simulink model "c00003M_harness"  (R2018a)
settings: Solver=FixedStepAuto  StartTime=0.0  StopTime=300  FixedStep=0.1  RelTol=1e-3
undefined symbols (not defined in the file): A1, hmax, PriorityTank, R1, R2, sigbuilder_block
(part 6 of 44)

== system c00003M_harness/M062 ==
  note: VALUES
      | ---------------------------------
      | ControlType = 1 | 2 | 3
      | FillTank = 0 | 1
      | EmptyTank = 0 | 1
      | ManualReference between 0 and 1
      | Tempreature between 0 and 100
      | EmergencyButton = 0 | 1
      | LiquidLevel between 0 and 1 (hmax)
  note: Inputs For Tank2
  note: NAMES
      | --------------------------------------------
      | CT1 = ControlType Tank 1
      | F1 = Fill Tank 1
      | E1 = Empty Tank 1
      | MR1 = Manual Reference Tank1
      | T1 = Temperature Tank 1
      | EB1 = Emergency Button Tank 1
      | LL1 = Liquid Level 1
  note: Inputs For Tank3
  note: Inputs For Tank1
  CT1 : Inport
  F1 : Inport  Port=2
  E1 : Inport  Port=3
  MR1 : Inport  Port=4
  T1 : Inport  Port=5
  EB1 : Inport  Port=6
  CT2 : Inport  Port=7
  F2 : Inport  Port=8
  E2 : Inport  Port=9
  MR2 : Inport  Port=10
  T2 : Inport  Port=11
  EB2 : Inport  Port=12
  Tank1 : Subsystem
  Tank2 : Subsystem
  LL1 : Outport
  LL2 : Outport  Port=2
  wires:
  EB1/1 -> Tank1/6(EB1)
  Tank2/1(LL2) -> LL2/1, Tank1/7(LL2)
  EB2/1 -> Tank2/6(EB2)
  CT2/1 -> Tank2/1(CT2)
  MR1/1 -> Tank1/4(MR1)
  T1/1 -> Tank1/5(T1)
  Tank1/1(LL1) -> LL1/1, Tank2/7(LL1)
  F2/1 -> Tank2/2(F2)
  E2/1 -> Tank2/3(E2)
  F1/1 -> Tank1/2(F1)
  E1/1 -> Tank1/3(E1)
  T2/1 -> Tank2/5(T2)
  CT1/1 -> Tank1/1(CT1)
  MR2/1 -> Tank2/4(MR2)

== system c00003M_harness/M063 ==
  note: VALUES
      | ---------------------------------
      | ControlType = 1 | 2 | 3
      | FillTank = 0 | 1
      | EmptyTank = 0 | 1
      | ManualReference between 0 and 1
      | Tempreature between 0 and 100
      | EmergencyButton = 0 | 1
      | LiquidLevel between 0 and 1 (hmax)
  note: Inputs For Tank2
  note: NAMES
      | --------------------------------------------
      | CT1 = ControlType Tank 1
      | F1 = Fill Tank 1
      | E1 = Empty Tank 1
      | MR1 = Manual Reference Tank1
      | T1 = Temperature Tank 1
      | EB1 = Emergency Button Tank 1
      | LL1 = Liquid Level 1
  note: Inputs For Tank3
  note: Inputs For Tank1
  CT1 : Inport
  F1 : Inport  Port=2
  E1 : Inport  Port=3
  MR1 : Inport  Port=4
  T1 : Inport  Port=5
  EB1 : Inport  Port=6
  CT2 : Inport  Port=7
  F2 : Inport  Port=8
  E2 : Inport  Port=9
  MR2 : Inport  Port=10
  T2 : Inport  Port=11
  EB2 : Inport  Port=12
  Tank1 : Subsystem
  Tank2 : Subsystem
  LL1 : Outport
  LL2 : Outport  Port=2
  wires:
  EB1/1 -> Tank1/6(EB1)
  Tank2/1(LL2) -> LL2/1, Tank1/7(LL2)
  EB2/1 -> Tank2/6(EB2)
  CT2/1 -> Tank2/1(CT2)
  MR1/1 -> Tank1/4(MR1)
  T1/1 -> Tank1/5(T1)
  Tank1/1(LL1) -> LL1/1, Tank2/7(LL1)
  F2/1 -> Tank2/2(F2)
  E2/1 -> Tank2/3(E2)
  F1/1 -> Tank1/2(F1)
  E1/1 -> Tank1/3(E1)
  T2/1 -> Tank2/5(T2)
  CT1/1 -> Tank1/1(CT1)
  MR2/1 -> Tank2/4(MR2)

== system c00003M_harness/M064 ==
  note: VALUES
      | ---------------------------------
      | ControlType = 1 | 2 | 3
      | FillTank = 0 | 1
      | EmptyTank = 0 | 1
      | ManualReference between 0 and 1
      | Tempreature between 0 and 100
      | EmergencyButton = 0 | 1
      | LiquidLevel between 0 and 1 (hmax)
  note: Inputs For Tank2
  note: NAMES
      | --------------------------------------------
      | CT1 = ControlType Tank 1
      | F1 = Fill Tank 1
      | E1 = Empty Tank 1
      | MR1 = Manual Reference Tank1
      | T1 = Temperature Tank 1
      | EB1 = Emergency Button Tank 1
      | LL1 = Liquid Level 1
  note: Inputs For Tank3
  note: Inputs For Tank1
  CT1 : Inport
  F1 : Inport  Port=2
  E1 : Inport  Port=3
  MR1 : Inport  Port=4
  T1 : Inport  Port=5
  EB1 : Inport  Port=6
  CT2 : Inport  Port=7
  F2 : Inport  Port=8
  E2 : Inport  Port=9
  MR2 : Inport  Port=10
  T2 : Inport  Port=11
  EB2 : Inport  Port=12
  Tank1 : Subsystem
  Tank2 : Subsystem
  LL1 : Outport
  LL2 : Outport  Port=2
  wires:
  EB1/1 -> Tank1/6(EB1)
  Tank2/1(LL2) -> LL2/1, Tank1/7(LL2)
  EB2/1 -> Tank2/6(EB2)
  CT2/1 -> Tank2/1(CT2)
  MR1/1 -> Tank1/4(MR1)
  T1/1 -> Tank1/5(T1)
  Tank1/1(LL1) -> LL1/1, Tank2/7(LL1)
  F2/1 -> Tank2/2(F2)
  E2/1 -> Tank2/3(E2)
  F1/1 -> Tank1/2(F1)
  E1/1 -> Tank1/3(E1)
  T2/1 -> Tank2/5(T2)
  CT1/1 -> Tank1/1(CT1)
  MR2/1 -> Tank2/4(MR2)

== system c00003M_harness/M065 ==
  note: VALUES
      | ---------------------------------
      | ControlType = 1 | 2 | 3
      | FillTank = 0 | 1
      | EmptyTank = 0 | 1
      | ManualReference between 0 and 1
      | Tempreature between 0 and 100
      | EmergencyButton = 0 | 1
      | LiquidLevel between 0 and 1 (hmax)
  note: Inputs For Tank2
  note: NAMES
      | --------------------------------------------
      | CT1 = ControlType Tank 1
      | F1 = Fill Tank 1
      | E1 = Empty Tank 1
      | MR1 = Manual Reference Tank1
      | T1 = Temperature Tank 1
      | EB1 = Emergency Button Tank 1
      | LL1 = Liquid Level 1
  note: Inputs For Tank3
  note: Inputs For Tank1
  CT1 : Inport
  F1 : Inport  Port=2
  E1 : Inport  Port=3
  MR1 : Inport  Port=4
  T1 : Inport  Port=5
  EB1 : Inport  Port=6
  CT2 : Inport  Port=7
  F2 : Inport  Port=8
  E2 : Inport  Port=9
  MR2 : Inport  Port=10
  T2 : Inport  Port=11
  EB2 : Inport  Port=12
  Tank1 : Subsystem
  Tank2 : Subsystem
  LL1 : Outport
  LL2 : Outport  Port=2
  wires:
  EB1/1 -> Tank1/6(EB1)
  Tank2/1(LL2) -> LL2/1, Tank1/7(LL2)
  EB2/1 -> Tank2/6(EB2)
  CT2/1 -> Tank2/1(CT2)
  MR1/1 -> Tank1/4(MR1)
  T1/1 -> Tank1/5(T1)
  Tank1/1(LL1) -> LL1/1, Tank2/7(LL1)
  F2/1 -> Tank2/2(F2)
  E2/1 -> Tank2/3(E2)
  F1/1 -> Tank1/2(F1)
  E1/1 -> Tank1/3(E1)
  T2/1 -> Tank2/5(T2)
  CT1/1 -> Tank1/1(CT1)
  MR2/1 -> Tank2/4(MR2)

== system c00003M_harness/M066 ==
  note: VALUES
      | ---------------------------------
      | ControlType = 1 | 2 | 3
      | FillTank = 0 | 1
      | EmptyTank = 0 | 1
      | ManualReference between 0 and 1
      | Tempreature between 0 and 100
      | EmergencyButton = 0 | 1
      | LiquidLevel between 0 and 1 (hmax)
  note: Inputs For Tank2
  note: NAMES
      | --------------------------------------------
      | CT1 = ControlType Tank 1
      | F1 = Fill Tank 1
      | E1 = Empty Tank 1
      | MR1 = Manual Reference Tank1
      | T1 = Temperature Tank 1
      | EB1 = Emergency Button Tank 1
      | LL1 = Liquid Level 1
  note: Inputs For Tank3
  note: Inputs For Tank1
  CT1 : Inport
  F1 : Inport  Port=2
  E1 : Inport  Port=3
  MR1 : Inport  Port=4
  T1 : Inport  Port=5
  EB1 : Inport  Port=6
  CT2 : Inport  Port=7
  F2 : Inport  Port=8
  E2 : Inport  Port=9
  MR2 : Inport  Port=10
  T2 : Inport  Port=11
  EB2 : Inport  Port=12
  Tank1 : Subsystem
  Tank2 : Subsystem
  LL1 : Outport
  LL2 : Outport  Port=2
  wires:
  EB1/1 -> Tank1/6(EB1)
  Tank2/1(LL2) -> LL2/1, Tank1/7(LL2)
  EB2/1 -> Tank2/6(EB2)
  CT2/1 -> Tank2/1(CT2)
  MR1/1 -> Tank1/4(MR1)
  T1/1 -> Tank1/5(T1)
  Tank1/1(LL1) -> LL1/1, Tank2/7(LL1)
  F2/1 -> Tank2/2(F2)
  E2/1 -> Tank2/3(E2)
  F1/1 -> Tank1/2(F1)
  E1/1 -> Tank1/3(E1)
  T2/1 -> Tank2/5(T2)
  CT1/1 -> Tank1/1(CT1)
  MR2/1 -> Tank2/4(MR2)

== system c00003M_harness/M067 ==
  note: VALUES
      | ---------------------------------
      | ControlType = 1 | 2 | 3
      | FillTank = 0 | 1
      | EmptyTank = 0 | 1
      | ManualReference between 0 and 1
      | Tempreature between 0 and 100
      | EmergencyButton = 0 | 1
      | LiquidLevel between 0 and 1 (hmax)
  note: Inputs For Tank2
  note: NAMES
      | --------------------------------------------
      | CT1 = ControlType Tank 1
      | F1 = Fill Tank 1
      | E1 = Empty Tank 1
      | MR1 = Manual Reference Tank1
      | T1 = Temperature Tank 1
      | EB1 = Emergency Button Tank 1
      | LL1 = Liquid Level 1
  note: Inputs For Tank3
  note: Inputs For Tank1
  CT1 : Inport
  F1 : Inport  Port=2
  E1 : Inport  Port=3
  MR1 : Inport  Port=4
  T1 : Inport  Port=5
  EB1 : Inport  Port=6
  CT2 : Inport  Port=7
  F2 : Inport  Port=8
  E2 : Inport  Port=9
  MR2 : Inport  Port=10
  T2 : Inport  Port=11
  EB2 : Inport  Port=12
  Tank1 : Subsystem
  Tank2 : Subsystem
  LL1 : Outport
  LL2 : Outport  Port=2
  wires:
  EB1/1 -> Tank1/6(EB1)
  Tank2/1(LL2) -> LL2/1, Tank1/7(LL2)
  EB2/1 -> Tank2/6(EB2)
  CT2/1 -> Tank2/1(CT2)
  MR1/1 -> Tank1/4(MR1)
  T1/1 -> Tank1/5(T1)
  Tank1/1(LL1) -> LL1/1, Tank2/7(LL1)
  F2/1 -> Tank2/2(F2)
  E2/1 -> Tank2/3(E2)
  F1/1 -> Tank1/2(F1)
  E1/1 -> Tank1/3(E1)
  T2/1 -> Tank2/5(T2)
  CT1/1 -> Tank1/1(CT1)
  MR2/1 -> Tank2/4(MR2)

== system c00003M_harness/M068 ==
  note: VALUES
      | ---------------------------------
      | ControlType = 1 | 2 | 3
      | FillTank = 0 | 1
      | EmptyTank = 0 | 1
      | ManualReference between 0 and 1
      | Tempreature between 0 and 100
      | EmergencyButton = 0 | 1
      | LiquidLevel between 0 and 1 (hmax)
  note: Inputs For Tank2
  note: NAMES
      | --------------------------------------------
      | CT1 = ControlType Tank 1
      | F1 = Fill Tank 1
      | E1 = Empty Tank 1
      | MR1 = Manual Reference Tank1
      | T1 = Temperature Tank 1
      | EB1 = Emergency Button Tank 1
      | LL1 = Liquid Level 1
  note: Inputs For Tank3
  note: Inputs For Tank1
  CT1 : Inport
  F1 : Inport  Port=2
  E1 : Inport  Port=3
  MR1 : Inport  Port=4
  T1 : Inport  Port=5
  EB1 : Inport  Port=6
  CT2 : Inport  Port=7
  F2 : Inport  Port=8
  E2 : Inport  Port=9
  MR2 : Inport  Port=10
  T2 : Inport  Port=11
  EB2 : Inport  Port=12
  Tank1 : Subsystem
  Tank2 : Subsystem
  LL1 : Outport
  LL2 : Outport  Port=2
  wires:
  EB1/1 -> Tank1/6(EB1)
  Tank2/1(LL2) -> LL2/1, Tank1/7(LL2)
  EB2/1 -> Tank2/6(EB2)
  CT2/1 -> Tank2/1(CT2)
  MR1/1 -> Tank1/4(MR1)
  T1/1 -> Tank1/5(T1)
  Tank1/1(LL1) -> LL1/1, Tank2/7(LL1)
  F2/1 -> Tank2/2(F2)
  E2/1 -> Tank2/3(E2)
  F1/1 -> Tank1/2(F1)
  E1/1 -> Tank1/3(E1)
  T2/1 -> Tank2/5(T2)
  CT1/1 -> Tank1/1(CT1)
  MR2/1 -> Tank2/4(MR2)

== system c00003M_harness/M069 ==
  note: VALUES
      | ---------------------------------
      | ControlType = 1 | 2 | 3
      | FillTank = 0 | 1
      | EmptyTank = 0 | 1
      | ManualReference between 0 and 1
      | Tempreature between 0 and 100
      | EmergencyButton = 0 | 1
      | LiquidLevel between 0 and 1 (hmax)
  note: Inputs For Tank2
  note: NAMES
      | --------------------------------------------
      | CT1 = ControlType Tank 1
      | F1 = Fill Tank 1
      | E1 = Empty Tank 1
      | MR1 = Manual Reference Tank1
      | T1 = Temperature Tank 1
      | EB1 = Emergency Button Tank 1
      | LL1 = Liquid Level 1
  note: Inputs For Tank3
  note: Inputs For Tank1
  CT1 : Inport
  F1 : Inport  Port=2
  E1 : Inport  Port=3
  MR1 : Inport  Port=4
  T1 : Inport  Port=5
  EB1 : Inport  Port=6
  CT2 : Inport  Port=7
  F2 : Inport  Port=8
  E2 : Inport  Port=9
  MR2 : Inport  Port=10
  T2 : Inport  Port=11
  EB2 : Inport  Port=12
  Tank1 : Subsystem
  Tank2 : Subsystem
  LL1 : Outport
  LL2 : Outport  Port=2
  wires:
  EB1/1 -> Tank1/6(EB1)
  Tank2/1(LL2) -> LL2/1, Tank1/7(LL2)
  EB2/1 -> Tank2/6(EB2)
  CT2/1 -> Tank2/1(CT2)
  MR1/1 -> Tank1/4(MR1)
  T1/1 -> Tank1/5(T1)
  Tank1/1(LL1) -> LL1/1, Tank2/7(LL1)
  F2/1 -> Tank2/2(F2)
  E2/1 -> Tank2/3(E2)
  F1/1 -> Tank1/2(F1)
  E1/1 -> Tank1/3(E1)
  T2/1 -> Tank2/5(T2)
  CT1/1 -> Tank1/1(CT1)
  MR2/1 -> Tank2/4(MR2)

== system c00003M_harness/M070 ==
  note: VALUES
      | ---------------------------------
      | ControlType = 1 | 2 | 3
      | FillTank = 0 | 1
      | EmptyTank = 0 | 1
      | ManualReference between 0 and 1
      | Tempreature between 0 and 100
      | EmergencyButton = 0 | 1
      | LiquidLevel between 0 and 1 (hmax)
  note: Inputs For Tank2
  note: NAMES
      | --------------------------------------------
      | CT1 = ControlType Tank 1
      | F1 = Fill Tank 1
      | E1 = Empty Tank 1
      | MR1 = Manual Reference Tank1
      | T1 = Temperature Tank 1
      | EB1 = Emergency Button Tank 1
      | LL1 = Liquid Level 1
  note: Inputs For Tank3
  note: Inputs For Tank1
  CT1 : Inport
  F1 : Inport  Port=2
  E1 : Inport  Port=3
  MR1 : Inport  Port=4
  T1 : Inport  Port=5
  EB1 : Inport  Port=6
  CT2 : Inport  Port=7
  F2 : Inport  Port=8
  E2 : Inport  Port=9
  MR2 : Inport  Port=10
  T2 : Inport  Port=11
  EB2 : Inport  Port=12
  Tank1 : Subsystem
  Tank2 : Subsystem
  LL1 : Outport
  LL2 : Outport  Port=2
  wires:
  EB1/1 -> Tank1/6(EB1)
  Tank2/1(LL2) -> LL2/1, Tank1/7(LL2)
  EB2/1 -> Tank2/6(EB2)
  CT2/1 -> Tank2/1(CT2)
  MR1/1 -> Tank1/4(MR1)
  T1/1 -> Tank1/5(T1)
  Tank1/1(LL1) -> LL1/1, Tank2/7(LL1)
  F2/1 -> Tank2/2(F2)
  E2/1 -> Tank2/3(E2)
  F1/1 -> Tank1/2(F1)
  E1/1 -> Tank1/3(E1)
  T2/1 -> Tank2/5(T2)
  CT1/1 -> Tank1/1(CT1)
  MR2/1 -> Tank2/4(MR2)

== system c00003M_harness/M071 ==
  note: VALUES
      | ---------------------------------
      | ControlType = 1 | 2 | 3
      | FillTank = 0 | 1
      | EmptyTank = 0 | 1
      | ManualReference between 0 and 1
      | Tempreature between 0 and 100
      | EmergencyButton = 0 | 1
      | LiquidLevel between 0 and 1 (hmax)
  note: Inputs For Tank2
  note: NAMES
      | --------------------------------------------
      | CT1 = ControlType Tank 1
      | F1 = Fill Tank 1
      | E1 = Empty Tank 1
      | MR1 = Manual Reference Tank1
      | T1 = Temperature Tank 1
      | EB1 = Emergency Button Tank 1
      | LL1 = Liquid Level 1
  note: Inputs For Tank3
  note: Inputs For Tank1
  CT1 : Inport
  F1 : Inport  Port=2
  E1 : Inport  Port=3
  MR1 : Inport  Port=4
  T1 : Inport  Port=5
  EB1 : Inport  Port=6
  CT2 : Inport  Port=7
  F2 : Inport  Port=8
  E2 : Inport  Port=9
  MR2 : Inport  Port=10
  T2 : Inport  Port=11
  EB2 : Inport  Port=12
  Tank1 : Subsystem
  Tank2 : Subsystem
  LL1 : Outport
  LL2 : Outport  Port=2
  wires:
  EB1/1 -> Tank1/6(EB1)
  Tank2/1(LL2) -> LL2/1, Tank1/7(LL2)
  EB2/1 -> Tank2/6(EB2)
  CT2/1 -> Tank2/1(CT2)
  MR1/1 -> Tank1/4(MR1)
  T1/1 -> Tank1/5(T1)
  Tank1/1(LL1) -> LL1/1, Tank2/7(LL1)
  F2/1 -> Tank2/2(F2)
  E2/1 -> Tank2/3(E2)
  F1/1 -> Tank1/2(F1)
  E1/1 -> Tank1/3(E1)
  T2/1 -> Tank2/5(T2)
  CT1/1 -> Tank1/1(CT1)
  MR2/1 -> Tank2/4(MR2)

== system c00003M_harness/M072 ==
  note: VALUES
      | ---------------------------------
      | ControlType = 1 | 2 | 3
      | FillTank = 0 | 1
      | EmptyTank = 0 | 1
      | ManualReference between 0 and 1
      | Tempreature between 0 and 100
      | EmergencyButton = 0 | 1
      | LiquidLevel between 0 and 1 (hmax)
  note: Inputs For Tank2
  note: NAMES
      | --------------------------------------------
      | CT1 = ControlType Tank 1
      | F1 = Fill Tank 1
      | E1 = Empty Tank 1
      | MR1 = Manual Reference Tank1
      | T1 = Temperature Tank 1
      | EB1 = Emergency Button Tank 1
      | LL1 = Liquid Level 1
  note: Inputs For Tank3
  note: Inputs For Tank1
  CT1 : Inport
  F1 : Inport  Port=2
  E1 : Inport  Port=3
  MR1 : Inport  Port=4
  T1 : Inport  Port=5
  EB1 : Inport  Port=6
  CT2 : Inport  Port=7
  F2 : Inport  Port=8
  E2 : Inport  Port=9
  MR2 : Inport  Port=10
  T2 : Inport  Port=11
  EB2 : Inport  Port=12
  Tank1 : Subsystem
  Tank2 : Subsystem
  LL1 : Outport
  LL2 : Outport  Port=2
  wires:
  EB1/1 -> Tank1/6(EB1)
  Tank2/1(LL2) -> LL2/1, Tank1/7(LL2)
  EB2/1 -> Tank2/6(EB2)
  CT2/1 -> Tank2/1(CT2)
  MR1/1 -> Tank1/4(MR1)
  T1/1 -> Tank1/5(T1)
  Tank1/1(LL1) -> LL1/1, Tank2/7(LL1)
  F2/1 -> Tank2/2(F2)
  E2/1 -> Tank2/3(E2)
  F1/1 -> Tank1/2(F1)
  E1/1 -> Tank1/3(E1)
  T2/1 -> Tank2/5(T2)
  CT1/1 -> Tank1/1(CT1)
  MR2/1 -> Tank2/4(MR2)

== system c00003M_harness/M073 ==
  note: VALUES
      | ---------------------------------
      | ControlType = 1 | 2 | 3
      | FillTank = 0 | 1
      | EmptyTank = 0 | 1
      | ManualReference between 0 and 1
      | Tempreature between 0 and 100
      | EmergencyButton = 0 | 1
      | LiquidLevel between 0 and 1 (hmax)
  note: Inputs For Tank2
  note: NAMES
      | --------------------------------------------
      | CT1 = ControlType Tank 1
      | F1 = Fill Tank 1
      | E1 = Empty Tank 1
      | MR1 = Manual Reference Tank1
      | T1 = Temperature Tank 1
      | EB1 = Emergency Button Tank 1
      | LL1 = Liquid Level 1
  note: Inputs For Tank3
  note: Inputs For Tank1
  CT1 : Inport
  F1 : Inport  Port=2
  E1 : Inport  Port=3
  MR1 : Inport  Port=4
  T1 : Inport  Port=5
  EB1 : Inport  Port=6
  CT2 : Inport  Port=7
  F2 : Inport  Port=8
  E2 : Inport  Port=9
  MR2 : Inport  Port=10
  T2 : Inport  Port=11
  EB2 : Inport  Port=12
  Tank1 : Subsystem
  Tank2 : Subsystem
  LL1 : Outport
  LL2 : Outport  Port=2
  wires:
  EB1/1 -> Tank1/6(EB1)
  Tank2/1(LL2) -> LL2/1, Tank1/7(LL2)
  EB2/1 -> Tank2/6(EB2)
  CT2/1 -> Tank2/1(CT2)
  MR1/1 -> Tank1/4(MR1)
  T1/1 -> Tank1/5(T1)
  Tank1/1(LL1) -> LL1/1, Tank2/7(LL1)
  F2/1 -> Tank2/2(F2)
  E2/1 -> Tank2/3(E2)
  F1/1 -> Tank1/2(F1)
  E1/1 -> Tank1/3(E1)
  T2/1 -> Tank2/5(T2)
  CT1/1 -> Tank1/1(CT1)
  MR2/1 -> Tank2/4(MR2)

== system c00003M_harness/M074 ==
  note: VALUES
      | ---------------------------------
      | ControlType = 1 | 2 | 3
      | FillTank = 0 | 1
      | EmptyTank = 0 | 1
      | ManualReference between 0 and 1
      | Tempreature between 0 and 100
      | EmergencyButton = 0 | 1
      | LiquidLevel between 0 and 1 (hmax)
  note: Inputs For Tank2
  note: NAMES
      | --------------------------------------------
      | CT1 = ControlType Tank 1
      | F1 = Fill Tank 1
      | E1 = Empty Tank 1
      | MR1 = Manual Reference Tank1
      | T1 = Temperature Tank 1
      | EB1 = Emergency Button Tank 1
      | LL1 = Liquid Level 1
  note: Inputs For Tank3
  note: Inputs For Tank1
  CT1 : Inport
  F1 : Inport  Port=2
  E1 : Inport  Port=3
  MR1 : Inport  Port=4
  T1 : Inport  Port=5
  EB1 : Inport  Port=6
  CT2 : Inport  Port=7
  F2 : Inport  Port=8
  E2 : Inport  Port=9
  MR2 : Inport  Port=10
  T2 : Inport  Port=11
  EB2 : Inport  Port=12
  Tank1 : Subsystem
  Tank2 : Subsystem
  LL1 : Outport
  LL2 : Outport  Port=2
  wires:
  EB1/1 -> Tank1/6(EB1)
  Tank2/1(LL2) -> LL2/1, Tank1/7(LL2)
  EB2/1 -> Tank2/6(EB2)
  CT2/1 -> Tank2/1(CT2)
  MR1/1 -> Tank1/4(MR1)
  T1/1 -> Tank1/5(T1)
  Tank1/1(LL1) -> LL1/1, Tank2/7(LL1)
  F2/1 -> Tank2/2(F2)
  E2/1 -> Tank2/3(E2)
  F1/1 -> Tank1/2(F1)
  E1/1 -> Tank1/3(E1)
  T2/1 -> Tank2/5(T2)
  CT1/1 -> Tank1/1(CT1)
  MR2/1 -> Tank2/4(MR2)

== system c00003M_harness/M075 ==
  note: VALUES
      | ---------------------------------
      | ControlType = 1 | 2 | 3
      | FillTank = 0 | 1
      | EmptyTank = 0 | 1
      | ManualReference between 0 and 1
      | Tempreature between 0 and 100
      | EmergencyButton = 0 | 1
      | LiquidLevel between 0 and 1 (hmax)
  note: Inputs For Tank2
  note: NAMES
      | --------------------------------------------
      | CT1 = ControlType Tank 1
      | F1 = Fill Tank 1
      | E1 = Empty Tank 1
      | MR1 = Manual Reference Tank1
      | T1 = Temperature Tank 1
      | EB1 = Emergency Button Tank 1
      | LL1 = Liquid Level 1
  note: Inputs For Tank3
  note: Inputs For Tank1
  CT1 : Inport
  F1 : Inport  Port=2
  E1 : Inport  Port=3
  MR1 : Inport  Port=4
  T1 : Inport  Port=5
  EB1 : Inport  Port=6
  CT2 : Inport  Port=7
  F2 : Inport  Port=8
  E2 : Inport  Port=9
  MR2 : Inport  Port=10
  T2 : Inport  Port=11
  EB2 : Inport  Port=12
  Tank1 : Subsystem
  Tank2 : Subsystem
  LL1 : Outport
  LL2 : Outport  Port=2
  wires:
  EB1/1 -> Tank1/6(EB1)
  Tank2/1(LL2) -> LL2/1, Tank1/7(LL2)
  EB2/1 -> Tank2/6(EB2)
  CT2/1 -> Tank2/1(CT2)
  MR1/1 -> Tank1/4(MR1)
  T1/1 -> Tank1/5(T1)
  Tank1/1(LL1) -> LL1/1, Tank2/7(LL1)
  F2/1 -> Tank2/2(F2)
  E2/1 -> Tank2/3(E2)
  F1/1 -> Tank1/2(F1)
  E1/1 -> Tank1/3(E1)
  T2/1 -> Tank2/5(T2)
  CT1/1 -> Tank1/1(CT1)
  MR2/1 -> Tank2/4(MR2)

== system c00003M_harness/M076 ==
  note: VALUES
      | ---------------------------------
      | ControlType = 1 | 2 | 3
      | FillTank = 0 | 1
      | EmptyTank = 0 | 1
      | ManualReference between 0 and 1
      | Tempreature between 0 and 100
      | EmergencyButton = 0 | 1
      | LiquidLevel between 0 and 1 (hmax)
  note: Inputs For Tank2
  note: NAMES
      | --------------------------------------------
      | CT1 = ControlType Tank 1
      | F1 = Fill Tank 1
      | E1 = Empty Tank 1
      | MR1 = Manual Reference Tank1
      | T1 = Temperature Tank 1
      | EB1 = Emergency Button Tank 1
      | LL1 = Liquid Level 1
  note: Inputs For Tank3
  note: Inputs For Tank1
  CT1 : Inport
  F1 : Inport  Port=2
  E1 : Inport  Port=3
  MR1 : Inport  Port=4
  T1 : Inport  Port=5
  EB1 : Inport  Port=6
  CT2 : Inport  Port=7
  F2 : Inport  Port=8
  E2 : Inport  Port=9
  MR2 : Inport  Port=10
  T2 : Inport  Port=11
  EB2 : Inport  Port=12
  Tank1 : Subsystem
  Tank2 : Subsystem
  LL1 : Outport
  LL2 : Outport  Port=2
  wires:
  EB1/1 -> Tank1/6(EB1)
  Tank2/1(LL2) -> LL2/1, Tank1/7(LL2)
  EB2/1 -> Tank2/6(EB2)
  CT2/1 -> Tank2/1(CT2)
  MR1/1 -> Tank1/4(MR1)
  T1/1 -> Tank1/5(T1)
  Tank1/1(LL1) -> LL1/1, Tank2/7(LL1)
  F2/1 -> Tank2/2(F2)
  E2/1 -> Tank2/3(E2)
  F1/1 -> Tank1/2(F1)
  E1/1 -> Tank1/3(E1)
  T2/1 -> Tank2/5(T2)
  CT1/1 -> Tank1/1(CT1)
  MR2/1 -> Tank2/4(MR2)

== system c00003M_harness/M077 ==
  note: VALUES
      | ---------------------------------
      | ControlType = 1 | 2 | 3
      | FillTank = 0 | 1
      | EmptyTank = 0 | 1
      | ManualReference between 0 and 1
      | Tempreature between 0 and 100
      | EmergencyButton = 0 | 1
      | LiquidLevel between 0 and 1 (hmax)
  note: Inputs For Tank2
  note: NAMES
      | --------------------------------------------
      | CT1 = ControlType Tank 1
      | F1 = Fill Tank 1
      | E1 = Empty Tank 1
      | MR1 = Manual Reference Tank1
      | T1 = Temperature Tank 1
      | EB1 = Emergency Button Tank 1
      | LL1 = Liquid Level 1
  note: Inputs For Tank3
  note: Inputs For Tank1
  CT1 : Inport
  F1 : Inport  Port=2
  E1 : Inport  Port=3
  MR1 : Inport  Port=4
  T1 : Inport  Port=5
  EB1 : Inport  Port=6
  CT2 : Inport  Port=7
  F2 : Inport  Port=8
  E2 : Inport  Port=9
  MR2 : Inport  Port=10
  T2 : Inport  Port=11
  EB2 : Inport  Port=12
  Tank1 : Subsystem
  Tank2 : Subsystem
  LL1 : Outport
  LL2 : Outport  Port=2
  wires:
  EB1/1 -> Tank1/6(EB1)
  Tank2/1(LL2) -> LL2/1, Tank1/7(LL2)
  EB2/1 -> Tank2/6(EB2)
  CT2/1 -> Tank2/1(CT2)
  MR1/1 -> Tank1/4(MR1)
  T1/1 -> Tank1/5(T1)
  Tank1/1(LL1) -> LL1/1, Tank2/7(LL1)
  F2/1 -> Tank2/2(F2)
  E2/1 -> Tank2/3(E2)
  F1/1 -> Tank1/2(F1)
  E1/1 -> Tank1/3(E1)
  T2/1 -> Tank2/5(T2)
  CT1/1 -> Tank1/1(CT1)
  MR2/1 -> Tank2/4(MR2)

== system c00003M_harness/M078 ==
  note: VALUES
      | ---------------------------------
      | ControlType = 1 | 2 | 3
      | FillTank = 0 | 1
      | EmptyTank = 0 | 1
      | ManualReference between 0 and 1
      | Tempreature between 0 and 100
      | EmergencyButton = 0 | 1
      | LiquidLevel between 0 and 1 (hmax)
  note: Inputs For Tank2
  note: NAMES
      | --------------------------------------------
      | CT1 = ControlType Tank 1
      | F1 = Fill Tank 1
      | E1 = Empty Tank 1
      | MR1 = Manual Reference Tank1
      | T1 = Temperature Tank 1
      | EB1 = Emergency Button Tank 1
      | LL1 = Liquid Level 1
  note: Inputs For Tank3
  note: Inputs For Tank1
  CT1 : Inport
  F1 : Inport  Port=2
  E1 : Inport  Port=3
  MR1 : Inport  Port=4
  T1 : Inport  Port=5
  EB1 : Inport  Port=6
  CT2 : Inport  Port=7
  F2 : Inport  Port=8
  E2 : Inport  Port=9
  MR2 : Inport  Port=10
  T2 : Inport  Port=11
  EB2 : Inport  Port=12
  Tank1 : Subsystem
  Tank2 : Subsystem
  LL1 : Outport
  LL2 : Outport  Port=2
  wires:
  EB1/1 -> Tank1/6(EB1)
  Tank2/1(LL2) -> LL2/1, Tank1/7(LL2)
  EB2/1 -> Tank2/6(EB2)
  CT2/1 -> Tank2/1(CT2)
  MR1/1 -> Tank1/4(MR1)
  T1/1 -> Tank1/5(T1)
  Tank1/1(LL1) -> LL1/1, Tank2/7(LL1)
  F2/1 -> Tank2/2(F2)
  E2/1 -> Tank2/3(E2)
  F1/1 -> Tank1/2(F1)
  E1/1 -> Tank1/3(E1)
  T2/1 -> Tank2/5(T2)
  CT1/1 -> Tank1/1(CT1)
  MR2/1 -> Tank2/4(MR2)

== system c00003M_harness/M079 ==
  note: VALUES
      | ---------------------------------
      | ControlType = 1 | 2 | 3
      | FillTank = 0 | 1
      | EmptyTank = 0 | 1
      | ManualReference between 0 and 1
      | Tempreature between 0 and 100
      | EmergencyButton = 0 | 1
      | LiquidLevel between 0 and 1 (hmax)
  note: Inputs For Tank2
  note: NAMES
      | --------------------------------------------
      | CT1 = ControlType Tank 1
      | F1 = Fill Tank 1
      | E1 = Empty Tank 1
      | MR1 = Manual Reference Tank1
      | T1 = Temperature Tank 1
      | EB1 = Emergency Button Tank 1
      | LL1 = Liquid Level 1
  note: Inputs For Tank3
  note: Inputs For Tank1
  CT1 : Inport
  F1 : Inport  Port=2
  E1 : Inport  Port=3
  MR1 : Inport  Port=4
  T1 : Inport  Port=5
  EB1 : Inport  Port=6
  CT2 : Inport  Port=7
  F2 : Inport  Port=8
  E2 : Inport  Port=9
  MR2 : Inport  Port=10
  T2 : Inport  Port=11
  EB2 : Inport  Port=12
  Tank1 : Subsystem
  Tank2 : Subsystem
  LL1 : Outport
  LL2 : Outport  Port=2
  wires:
  EB1/1 -> Tank1/6(EB1)
  Tank2/1(LL2) -> LL2/1, Tank1/7(LL2)
  EB2/1 -> Tank2/6(EB2)
  CT2/1 -> Tank2/1(CT2)
  MR1/1 -> Tank1/4(MR1)
  T1/1 -> Tank1/5(T1)
  Tank1/1(LL1) -> LL1/1, Tank2/7(LL1)
  F2/1 -> Tank2/2(F2)
  E2/1 -> Tank2/3(E2)
  F1/1 -> Tank1/2(F1)
  E1/1 -> Tank1/3(E1)
  T2/1 -> Tank2/5(T2)
  CT1/1 -> Tank1/1(CT1)
  MR2/1 -> Tank2/4(MR2)

== system c00003M_harness/M080 ==
  note: VALUES
      | ---------------------------------
      | ControlType = 1 | 2 | 3
      | FillTank = 0 | 1
      | EmptyTank = 0 | 1
      | ManualReference between 0 and 1
      | Tempreature between 0 and 100
      | EmergencyButton = 0 | 1
      | LiquidLevel between 0 and 1 (hmax)
  note: Inputs For Tank2
  note: NAMES
      | --------------------------------------------
      | CT1 = ControlType Tank 1
      | F1 = Fill Tank 1
      | E1 = Empty Tank 1
      | MR1 = Manual Reference Tank1
      | T1 = Temperature Tank 1
      | EB1 = Emergency Button Tank 1
      | LL1 = Liquid Level 1
  note: Inputs For Tank3
  note: Inputs For Tank1
  CT1 : Inport
  F1 : Inport  Port=2
  E1 : Inport  Port=3
  MR1 : Inport  Port=4
  T1 : Inport  Port=5
  EB1 : Inport  Port=6
  CT2 : Inport  Port=7
  F2 : Inport  Port=8
  E2 : Inport  Port=9
  MR2 : Inport  Port=10
  T2 : Inport  Port=11
  EB2 : Inport  Port=12
  Tank1 : Subsystem
  Tank2 : Subsystem
  LL1 : Outport
  LL2 : Outport  Port=2
  wires:
  EB1/1 -> Tank1/6(EB1)
  Tank2/1(LL2) -> LL2/1, Tank1/7(LL2)
  EB2/1 -> Tank2/6(EB2)
  CT2/1 -> Tank2/1(CT2)
  MR1/1 -> Tank1/4(MR1)
  T1/1 -> Tank1/5(T1)
  Tank1/1(LL1) -> LL1/1, Tank2/7(LL1)
  F2/1 -> Tank2/2(F2)
  E2/1 -> Tank2/3(E2)
  F1/1 -> Tank1/2(F1)
  E1/1 -> Tank1/3(E1)
  T2/1 -> Tank2/5(T2)
  CT1/1 -> Tank1/1(CT1)
  MR2/1 -> Tank2/4(MR2)

== system c00003M_harness/M081 ==
  note: VALUES
      | ---------------------------------
      | ControlType = 1 | 2 | 3
      | FillTank = 0 | 1
      | EmptyTank = 0 | 1
      | ManualReference between 0 and 1
      | Tempreature between 0 and 100
      | EmergencyButton = 0 | 1
      | LiquidLevel between 0 and 1 (hmax)
  note: Inputs For Tank2
  note: NAMES
      | --------------------------------------------
      | CT1 = ControlType Tank 1
      | F1 = Fill Tank 1
      | E1 = Empty Tank 1
      | MR1 = Manual Reference Tank1
      | T1 = Temperature Tank 1
      | EB1 = Emergency Button Tank 1
      | LL1 = Liquid Level 1
  note: Inputs For Tank3
  note: Inputs For Tank1
  CT1 : Inport
  F1 : Inport  Port=2
  E1 : Inport  Port=3
  MR1 : Inport  Port=4
  T1 : Inport  Port=5
  EB1 : Inport  Port=6
  CT2 : Inport  Port=7
  F2 : Inport  Port=8
  E2 : Inport  Port=9
  MR2 : Inport  Port=10
  T2 : Inport  Port=11
  EB2 : Inport  Port=12
  Tank1 : Subsystem
  Tank2 : Subsystem
  LL1 : Outport
  LL2 : Outport  Port=2
  wires:
  EB1/1 -> Tank1/6(EB1)
  Tank2/1(LL2) -> LL2/1, Tank1/7(LL2)
  EB2/1 -> Tank2/6(EB2)
  CT2/1 -> Tank2/1(CT2)
  MR1/1 -> Tank1/4(MR1)
  T1/1 -> Tank1/5(T1)
  Tank1/1(LL1) -> LL1/1, Tank2/7(LL1)
  F2/1 -> Tank2/2(F2)
  E2/1 -> Tank2/3(E2)
  F1/1 -> Tank1/2(F1)
  E1/1 -> Tank1/3(E1)
  T2/1 -> Tank2/5(T2)
  CT1/1 -> Tank1/1(CT1)
  MR2/1 -> Tank2/4(MR2)

== system c00003M_harness/M082 ==
  note: VALUES
      | ---------------------------------
      | ControlType = 1 | 2 | 3
      | FillTank = 0 | 1
      | EmptyTank = 0 | 1
      | ManualReference between 0 and 1
      | Tempreature between 0 and 100
      | EmergencyButton = 0 | 1
      | LiquidLevel between 0 and 1 (hmax)
  note: Inputs For Tank2
  note: NAMES
      | --------------------------------------------
      | CT1 = ControlType Tank 1
      | F1 = Fill Tank 1
      | E1 = Empty Tank 1
      | MR1 = Manual Reference Tank1
      | T1 = Temperature Tank 1
      | EB1 = Emergency Button Tank 1
      | LL1 = Liquid Level 1
  note: Inputs For Tank3
  note: Inputs For Tank1
  CT1 : Inport
  F1 : Inport  Port=2
  E1 : Inport  Port=3
  MR1 : Inport  Port=4
  T1 : Inport  Port=5
  EB1 : Inport  Port=6
  CT2 : Inport  Port=7
  F2 : Inport  Port=8
  E2 : Inport  Port=9
  MR2 : Inport  Port=10
  T2 : Inport  Port=11
  EB2 : Inport  Port=12
  Tank1 : Subsystem
  Tank2 : Subsystem
  LL1 : Outport
  LL2 : Outport  Port=2
  wires:
  EB1/1 -> Tank1/6(EB1)
  Tank2/1(LL2) -> LL2/1, Tank1/7(LL2)
  EB2/1 -> Tank2/6(EB2)
  CT2/1 -> Tank2/1(CT2)
  MR1/1 -> Tank1/4(MR1)
  T1/1 -> Tank1/5(T1)
  Tank1/1(LL1) -> LL1/1, Tank2/7(LL1)
  F2/1 -> Tank2/2(F2)
  E2/1 -> Tank2/3(E2)
  F1/1 -> Tank1/2(F1)
  E1/1 -> Tank1/3(E1)
  T2/1 -> Tank2/5(T2)
  CT1/1 -> Tank1/1(CT1)
  MR2/1 -> Tank2/4(MR2)

== system c00003M_harness/M083 ==
  note: VALUES
      | ---------------------------------
      | ControlType = 1 | 2 | 3
      | FillTank = 0 | 1
      | EmptyTank = 0 | 1
      | ManualReference between 0 and 1
      | Tempreature between 0 and 100
      | EmergencyButton = 0 | 1
      | LiquidLevel between 0 and 1 (hmax)
  note: Inputs For Tank2
  note: NAMES
      | --------------------------------------------
      | CT1 = ControlType Tank 1
      | F1 = Fill Tank 1
      | E1 = Empty Tank 1
      | MR1 = Manual Reference Tank1
      | T1 = Temperature Tank 1
      | EB1 = Emergency Button Tank 1
      | LL1 = Liquid Level 1
  note: Inputs For Tank3
  note: Inputs For Tank1
  CT1 : Inport
  F1 : Inport  Port=2
  E1 : Inport  Port=3
  MR1 : Inport  Port=4
  T1 : Inport  Port=5
  EB1 : Inport  Port=6
  CT2 : Inport  Port=7
  F2 : Inport  Port=8
  E2 : Inport  Port=9
  MR2 : Inport  Port=10
  T2 : Inport  Port=11
  EB2 : Inport  Port=12
  Tank1 : Subsystem
  Tank2 : Subsystem
  LL1 : Outport
  LL2 : Outport  Port=2
  wires:
  EB1/1 -> Tank1/6(EB1)
  Tank2/1(LL2) -> LL2/1, Tank1/7(LL2)
  EB2/1 -> Tank2/6(EB2)
  CT2/1 -> Tank2/1(CT2)
  MR1/1 -> Tank1/4(MR1)
  T1/1 -> Tank1/5(T1)
  Tank1/1(LL1) -> LL1/1, Tank2/7(LL1)
  F2/1 -> Tank2/2(F2)
  E2/1 -> Tank2/3(E2)
  F1/1 -> Tank1/2(F1)
  E1/1 -> Tank1/3(E1)
  T2/1 -> Tank2/5(T2)
  CT1/1 -> Tank1/1(CT1)
  MR2/1 -> Tank2/4(MR2)

== system c00003M_harness/M118 ==
  note: VALUES
      | ---------------------------------
      | ControlType = 1 | 2 | 3
      | FillTank = 0 | 1
      | EmptyTank = 0 | 1
      | ManualReference between 0 and 1
      | Tempreature between 0 and 100
      | EmergencyButton = 0 | 1
      | LiquidLevel between 0 and 1 (hmax)
  note: Inputs For Tank2
  note: NAMES
      | --------------------------------------------
      | CT1 = ControlType Tank 1
      | F1 = Fill Tank 1
      | E1 = Empty Tank 1
      | MR1 = Manual Reference Tank1
      | T1 = Temperature Tank 1
      | EB1 = Emergency Button Tank 1
      | LL1 = Liquid Level 1
  note: Inputs For Tank3
  note: Inputs For Tank1
  CT1 : Inport
  F1 : Inport  Port=2
  E1 : Inport  Port=3
  MR1 : Inport  Port=4
  T1 : Inport  Port=5
  EB1 : Inport  Port=6
  CT2 : Inport  Port=7
  F2 : Inport  Port=8
  E2 : Inport  Port=9
  MR2 : Inport  Port=10
  T2 : Inport  Port=11
  EB2 : Inport  Port=12
  Tank1 : Subsystem
  Tank2 : Subsystem
  LL1 : Outport
  LL2 : Outport  Port=2
  wires:
  EB1/1 -> Tank1/6(EB1)
  Tank2/1(LL2) -> LL2/1, Tank1/7(LL2)
  EB2/1 -> Tank2/6(EB2)
  CT2/1 -> Tank2/1(CT2)
  MR1/1 -> Tank1/4(MR1)
  T1/1 -> Tank1/5(T1)
  Tank1/1(LL1) -> LL1/1, Tank2/7(LL1)
  F2/1 -> Tank2/2(F2)
  E2/1 -> Tank2/3(E2)
  F1/1 -> Tank1/2(F1)
  E1/1 -> Tank1/3(E1)
  T2/1 -> Tank2/5(T2)
  CT1/1 -> Tank1/1(CT1)
  MR2/1 -> Tank2/4(MR2)

== system c00003M_harness/M119 ==
  note: VALUES
      | ---------------------------------
      | ControlType = 1 | 2 | 3
      | FillTank = 0 | 1
      | EmptyTank = 0 | 1
      | ManualReference between 0 and 1
      | Tempreature between 0 and 100
      | EmergencyButton = 0 | 1
      | LiquidLevel between 0 and 1 (hmax)
  note: Inputs For Tank2
  note: NAMES
      | --------------------------------------------
      | CT1 = ControlType Tank 1
      | F1 = Fill Tank 1
      | E1 = Empty Tank 1
      | MR1 = Manual Reference Tank1
      | T1 = Temperature Tank 1
      | EB1 = Emergency Button Tank 1
      | LL1 = Liquid Level 1
  note: Inputs For Tank3
  note: Inputs For Tank1
  CT1 : Inport
  F1 : Inport  Port=2
  E1 : Inport  Port=3
  MR1 : Inport  Port=4
  T1 : Inport  Port=5
  EB1 : Inport  Port=6
  CT2 : Inport  Port=7
  F2 : Inport  Port=8
  E2 : Inport  Port=9
  MR2 : Inport  Port=10
  T2 : Inport  Port=11
  EB2 : Inport  Port=12
  Tank1 : Subsystem
  Tank2 : Subsystem
  LL1 : Outport
  LL2 : Outport  Port=2
  wires:
  EB1/1 -> Tank1/6(EB1)
  Tank2/1(LL2) -> LL2/1, Tank1/7(LL2)
  EB2/1 -> Tank2/6(EB2)
  CT2/1 -> Tank2/1(CT2)
  MR1/1 -> Tank1/4(MR1)
  T1/1 -> Tank1/5(T1)
  Tank1/1(LL1) -> LL1/1, Tank2/7(LL1)
  F2/1 -> Tank2/2(F2)
  E2/1 -> Tank2/3(E2)
  F1/1 -> Tank1/2(F1)
  E1/1 -> Tank1/3(E1)
  T2/1 -> Tank2/5(T2)
  CT1/1 -> Tank1/1(CT1)
  MR2/1 -> Tank2/4(MR2)

== system c00003M_harness/M120 ==
  note: VALUES
      | ---------------------------------
      | ControlType = 1 | 2 | 3
      | FillTank = 0 | 1
      | EmptyTank = 0 | 1
      | ManualReference between 0 and 1
      | Tempreature between 0 and 100
      | EmergencyButton = 0 | 1
      | LiquidLevel between 0 and 1 (hmax)
  note: Inputs For Tank2
  note: NAMES
      | --------------------------------------------
      | CT1 = ControlType Tank 1
      | F1 = Fill Tank 1
      | E1 = Empty Tank 1
      | MR1 = Manual Reference Tank1
      | T1 = Temperature Tank 1
      | EB1 = Emergency Button Tank 1
      | LL1 = Liquid Level 1
  note: Inputs For Tank3
  note: Inputs For Tank1
  CT1 : Inport
  F1 : Inport  Port=2
  E1 : Inport  Port=3
  MR1 : Inport  Port=4
  T1 : Inport  Port=5
  EB1 : Inport  Port=6
  CT2 : Inport  Port=7
  F2 : Inport  Port=8
  E2 : Inport  Port=9
  MR2 : Inport  Port=10
  T2 : Inport  Port=11
  EB2 : Inport  Port=12
  Tank1 : Subsystem
  Tank2 : Subsystem
  LL1 : Outport
  LL2 : Outport  Port=2
  wires:
  EB1/1 -> Tank1/6(EB1)
  Tank2/1(LL2) -> LL2/1, Tank1/7(LL2)
  EB2/1 -> Tank2/6(EB2)
  CT2/1 -> Tank2/1(CT2)
  MR1/1 -> Tank1/4(MR1)
  T1/1 -> Tank1/5(T1)
  Tank1/1(LL1) -> LL1/1, Tank2/7(LL1)
  F2/1 -> Tank2/2(F2)
  E2/1 -> Tank2/3(E2)
  F1/1 -> Tank1/2(F1)
  E1/1 -> Tank1/3(E1)
  T2/1 -> Tank2/5(T2)
  CT1/1 -> Tank1/1(CT1)
  MR2/1 -> Tank2/4(MR2)

== system c00003M_harness/M121 ==
  note: VALUES
      | ---------------------------------
      | ControlType = 1 | 2 | 3
      | FillTank = 0 | 1
      | EmptyTank = 0 | 1
      | ManualReference between 0 and 1
      | Tempreature between 0 and 100
      | EmergencyButton = 0 | 1
      | LiquidLevel between 0 and 1 (hmax)
  note: Inputs For Tank2
  note: NAMES
      | --------------------------------------------
      | CT1 = ControlType Tank 1
      | F1 = Fill Tank 1
      | E1 = Empty Tank 1
      | MR1 = Manual Reference Tank1
      | T1 = Temperature Tank 1
      | EB1 = Emergency Button Tank 1
      | LL1 = Liquid Level 1
  note: Inputs For Tank3
  note: Inputs For Tank1
  CT1 : Inport
  F1 : Inport  Port=2
  E1 : Inport  Port=3
  MR1 : Inport  Port=4
  T1 : Inport  Port=5
  EB1 : Inport  Port=6
  CT2 : Inport  Port=7
  F2 : Inport  Port=8
  E2 : Inport  Port=9
  MR2 : Inport  Port=10
  T2 : Inport  Port=11
  EB2 : Inport  Port=12
  Tank1 : Subsystem
  Tank2 : Subsystem
  LL1 : Outport
  LL2 : Outport  Port=2
  wires:
  EB1/1 -> Tank1/6(EB1)
  Tank2/1(LL2) -> LL2/1, Tank1/7(LL2)
  EB2/1 -> Tank2/6(EB2)
  CT2/1 -> Tank2/1(CT2)
  MR1/1 -> Tank1/4(MR1)
  T1/1 -> Tank1/5(T1)
  Tank1/1(LL1) -> LL1/1, Tank2/7(LL1)
  F2/1 -> Tank2/2(F2)
  E2/1 -> Tank2/3(E2)
  F1/1 -> Tank1/2(F1)
  E1/1 -> Tank1/3(E1)
  T2/1 -> Tank2/5(T2)
  CT1/1 -> Tank1/1(CT1)
  MR2/1 -> Tank2/4(MR2)

== system c00003M_harness/M122 ==
  note: VALUES
      | ---------------------------------
      | ControlType = 1 | 2 | 3
      | FillTank = 0 | 1
      | EmptyTank = 0 | 1
      | ManualReference between 0 and 1
      | Tempreature between 0 and 100
      | EmergencyButton = 0 | 1
      | LiquidLevel between 0 and 1 (hmax)
  note: Inputs For Tank2
  note: NAMES
      | --------------------------------------------
      | CT1 = ControlType Tank 1
      | F1 = Fill Tank 1
      | E1 = Empty Tank 1
      | MR1 = Manual Reference Tank1
      | T1 = Temperature Tank 1
      | EB1 = Emergency Button Tank 1
      | LL1 = Liquid Level 1
  note: Inputs For Tank3
  note: Inputs For Tank1
  CT1 : Inport
  F1 : Inport  Port=2
  E1 : Inport  Port=3
  MR1 : Inport  Port=4
  T1 : Inport  Port=5
  EB1 : Inport  Port=6
  CT2 : Inport  Port=7
  F2 : Inport  Port=8
  E2 : Inport  Port=9
  MR2 : Inport  Port=10
  T2 : Inport  Port=11
  EB2 : Inport  Port=12
  Tank1 : Subsystem
  Tank2 : Subsystem
  LL1 : Outport
  LL2 : Outport  Port=2
  wires:
  EB1/1 -> Tank1/6(EB1)
  Tank2/1(LL2) -> LL2/1, Tank1/7(LL2)
  EB2/1 -> Tank2/6(EB2)
  CT2/1 -> Tank2/1(CT2)
  MR1/1 -> Tank1/4(MR1)
  T1/1 -> Tank1/5(T1)
  Tank1/1(LL1) -> LL1/1, Tank2/7(LL1)
  F2/1 -> Tank2/2(F2)
  E2/1 -> Tank2/3(E2)
  F1/1 -> Tank1/2(F1)
  E1/1 -> Tank1/3(E1)
  T2/1 -> Tank2/5(T2)
  CT1/1 -> Tank1/1(CT1)
  MR2/1 -> Tank2/4(MR2)

== system c00003M_harness/M123 ==
  note: VALUES
      | ---------------------------------
      | ControlType = 1 | 2 | 3
      | FillTank = 0 | 1
      | EmptyTank = 0 | 1
      | ManualReference between 0 and 1
      | Tempreature between 0 and 100
      | EmergencyButton = 0 | 1
      | LiquidLevel between 0 and 1 (hmax)
  note: Inputs For Tank2
  note: NAMES
      | --------------------------------------------
      | CT1 = ControlType Tank 1
      | F1 = Fill Tank 1
      | E1 = Empty Tank 1
      | MR1 = Manual Reference Tank1
      | T1 = Temperature Tank 1
      | EB1 = Emergency Button Tank 1
      | LL1 = Liquid Level 1
  note: Inputs For Tank3
  note: Inputs For Tank1
  CT1 : Inport
  F1 : Inport  Port=2
  E1 : Inport  Port=3
  MR1 : Inport  Port=4
  T1 : Inport  Port=5
  EB1 : Inport  Port=6
  CT2 : Inport  Port=7
  F2 : Inport  Port=8
  E2 : Inport  Port=9
  MR2 : Inport  Port=10
  T2 : Inport  Port=11
  EB2 : Inport  Port=12
  Tank1 : Subsystem
  Tank2 : Subsystem
  LL1 : Outport
  LL2 : Outport  Port=2
  wires:
  EB1/1 -> Tank1/6(EB1)
  Tank2/1(LL2) -> LL2/1, Tank1/7(LL2)
  EB2/1 -> Tank2/6(EB2)
  CT2/1 -> Tank2/1(CT2)
  MR1/1 -> Tank1/4(MR1)
  T1/1 -> Tank1/5(T1)
  Tank1/1(LL1) -> LL1/1, Tank2/7(LL1)
  F2/1 -> Tank2/2(F2)
  E2/1 -> Tank2/3(E2)
  F1/1 -> Tank1/2(F1)
  E1/1 -> Tank1/3(E1)
  T2/1 -> Tank2/5(T2)
  CT1/1 -> Tank1/1(CT1)
  MR2/1 -> Tank2/4(MR2)

== system c00003M_harness/M124 ==
  note: VALUES
      | ---------------------------------
      | ControlType = 1 | 2 | 3
      | FillTank = 0 | 1
      | EmptyTank = 0 | 1
      | ManualReference between 0 and 1
      | Tempreature between 0 and 100
      | EmergencyButton = 0 | 1
      | LiquidLevel between 0 and 1 (hmax)
  note: Inputs For Tank2
  note: NAMES
      | --------------------------------------------
      | CT1 = ControlType Tank 1
      | F1 = Fill Tank 1
      | E1 = Empty Tank 1
      | MR1 = Manual Reference Tank1
      | T1 = Temperature Tank 1
      | EB1 = Emergency Button Tank 1
      | LL1 = Liquid Level 1
  note: Inputs For Tank3
  note: Inputs For Tank1
  CT1 : Inport
  F1 : Inport  Port=2
  E1 : Inport  Port=3
  MR1 : Inport  Port=4
  T1 : Inport  Port=5
  EB1 : Inport  Port=6
  CT2 : Inport  Port=7
  F2 : Inport  Port=8
  E2 : Inport  Port=9
  MR2 : Inport  Port=10
  T2 : Inport  Port=11
  EB2 : Inport  Port=12
  Tank1 : Subsystem
  Tank2 : Subsystem
  LL1 : Outport
  LL2 : Outport  Port=2
  wires:
  EB1/1 -> Tank1/6(EB1)
  Tank2/1(LL2) -> LL2/1, Tank1/7(LL2)
  EB2/1 -> Tank2/6(EB2)
  CT2/1 -> Tank2/1(CT2)
  MR1/1 -> Tank1/4(MR1)
  T1/1 -> Tank1/5(T1)
  Tank1/1(LL1) -> LL1/1, Tank2/7(LL1)
  F2/1 -> Tank2/2(F2)
  E2/1 -> Tank2/3(E2)
  F1/1 -> Tank1/2(F1)
  E1/1 -> Tank1/3(E1)
  T2/1 -> Tank2/5(T2)
  CT1/1 -> Tank1/1(CT1)
  MR2/1 -> Tank2/4(MR2)

== system c00003M_harness/M125 ==
  note: VALUES
      | ---------------------------------
      | ControlType = 1 | 2 | 3
      | FillTank = 0 | 1
      | EmptyTank = 0 | 1
      | ManualReference between 0 and 1
      | Tempreature between 0 and 100
      | EmergencyButton = 0 | 1
      | LiquidLevel between 0 and 1 (hmax)
  note: Inputs For Tank2
  note: NAMES
      | --------------------------------------------
      | CT1 = ControlType Tank 1
      | F1 = Fill Tank 1
      | E1 = Empty Tank 1
      | MR1 = Manual Reference Tank1
      | T1 = Temperature Tank 1
      | EB1 = Emergency Button Tank 1
      | LL1 = Liquid Level 1
  note: Inputs For Tank3
  note: Inputs For Tank1
  CT1 : Inport
  F1 : Inport  Port=2
  E1 : Inport  Port=3
  MR1 : Inport  Port=4
  T1 : Inport  Port=5
  EB1 : Inport  Port=6
  CT2 : Inport  Port=7
  F2 : Inport  Port=8
  E2 : Inport  Port=9
  MR2 : Inport  Port=10
  T2 : Inport  Port=11
  EB2 : Inport  Port=12
  Tank1 : Subsystem
  Tank2 : Subsystem
  LL1 : Outport
  LL2 : Outport  Port=2
  wires:
  EB1/1 -> Tank1/6(EB1)
  Tank2/1(LL2) -> LL2/1, Tank1/7(LL2)
  EB2/1 -> Tank2/6(EB2)
  CT2/1 -> Tank2/1(CT2)
  MR1/1 -> Tank1/4(MR1)
  T1/1 -> Tank1/5(T1)
  Tank1/1(LL1) -> LL1/1, Tank2/7(LL1)
  F2/1 -> Tank2/2(F2)
  E2/1 -> Tank2/3(E2)
  F1/1 -> Tank1/2(F1)
  E1/1 -> Tank1/3(E1)
  T2/1 -> Tank2/5(T2)
  CT1/1 -> Tank1/1(CT1)
  MR2/1 -> Tank2/4(MR2)

== system c00003M_harness/M126 ==
  note: VALUES
      | ---------------------------------
      | ControlType = 1 | 2 | 3
      | FillTank = 0 | 1
      | EmptyTank = 0 | 1
      | ManualReference between 0 and 1
      | Tempreature between 0 and 100
      | EmergencyButton = 0 | 1
      | LiquidLevel between 0 and 1 (hmax)
  note: Inputs For Tank2
  note: NAMES
      | --------------------------------------------
      | CT1 = ControlType Tank 1
      | F1 = Fill Tank 1
      | E1 = Empty Tank 1
      | MR1 = Manual Reference Tank1
      | T1 = Temperature Tank 1
      | EB1 = Emergency Button Tank 1
      | LL1 = Liquid Level 1
  note: Inputs For Tank3
  note: Inputs For Tank1
  CT1 : Inport
  F1 : Inport  Port=2
  E1 : Inport  Port=3
  MR1 : Inport  Port=4
  T1 : Inport  Port=5
  EB1 : Inport  Port=6
  CT2 : Inport  Port=7
  F2 : Inport  Port=8
  E2 : Inport  Port=9
  MR2 : Inport  Port=10
  T2 : Inport  Port=11
  EB2 : Inport  Port=12
  Tank1 : Subsystem
  Tank2 : Subsystem
  LL1 : Outport
  LL2 : Outport  Port=2
  wires:
  EB1/1 -> Tank1/6(EB1)
  Tank2/1(LL2) -> LL2/1, Tank1/7(LL2)
  EB2/1 -> Tank2/6(EB2)
  CT2/1 -> Tank2/1(CT2)
  MR1/1 -> Tank1/4(MR1)
  T1/1 -> Tank1/5(T1)
  Tank1/1(LL1) -> LL1/1, Tank2/7(LL1)
  F2/1 -> Tank2/2(F2)
  E2/1 -> Tank2/3(E2)
  F1/1 -> Tank1/2(F1)
  E1/1 -> Tank1/3(E1)
  T2/1 -> Tank2/5(T2)
  CT1/1 -> Tank1/1(CT1)
  MR2/1 -> Tank2/4(MR2)

== system c00003M_harness/M127 ==
  note: VALUES
      | ---------------------------------
      | ControlType = 1 | 2 | 3
      | FillTank = 0 | 1
      | EmptyTank = 0 | 1
      | ManualReference between 0 and 1
      | Tempreature between 0 and 100
      | EmergencyButton = 0 | 1
      | LiquidLevel between 0 and 1 (hmax)
  note: Inputs For Tank2
  note: NAMES
      | --------------------------------------------
      | CT1 = ControlType Tank 1
      | F1 = Fill Tank 1
      | E1 = Empty Tank 1
      | MR1 = Manual Reference Tank1
      | T1 = Temperature Tank 1
      | EB1 = Emergency Button Tank 1
      | LL1 = Liquid Level 1
  note: Inputs For Tank3
  note: Inputs For Tank1
  CT1 : Inport
  F1 : Inport  Port=2
  E1 : Inport  Port=3
  MR1 : Inport  Port=4
  T1 : Inport  Port=5
  EB1 : Inport  Port=6
  CT2 : Inport  Port=7
  F2 : Inport  Port=8
  E2 : Inport  Port=9
  MR2 : Inport  Port=10
  T2 : Inport  Port=11
  EB2 : Inport  Port=12
  Tank1 : Subsystem
  Tank2 : Subsystem
  LL1 : Outport
  LL2 : Outport  Port=2
  wires:
  EB1/1 -> Tank1/6(EB1)
  Tank2/1(LL2) -> LL2/1, Tank1/7(LL2)
  EB2/1 -> Tank2/6(EB2)
  CT2/1 -> Tank2/1(CT2)
  MR1/1 -> Tank1/4(MR1)
  T1/1 -> Tank1/5(T1)
  Tank1/1(LL1) -> LL1/1, Tank2/7(LL1)
  F2/1 -> Tank2/2(F2)
  E2/1 -> Tank2/3(E2)
  F1/1 -> Tank1/2(F1)
  E1/1 -> Tank1/3(E1)
  T2/1 -> Tank2/5(T2)
  CT1/1 -> Tank1/1(CT1)
  MR2/1 -> Tank2/4(MR2)

== system c00003M_harness/M128 ==
  note: VALUES
      | ---------------------------------
      | ControlType = 1 | 2 | 3
      | FillTank = 0 | 1
      | EmptyTank = 0 | 1
      | ManualReference between 0 and 1
      | Tempreature between 0 and 100
      | EmergencyButton = 0 | 1
      | LiquidLevel between 0 and 1 (hmax)
  note: Inputs For Tank2
  note: NAMES
      | --------------------------------------------
      | CT1 = ControlType Tank 1
      | F1 = Fill Tank 1
      | E1 = Empty Tank 1
      | MR1 = Manual Reference Tank1
      | T1 = Temperature Tank 1
      | EB1 = Emergency Button Tank 1
      | LL1 = Liquid Level 1
  note: Inputs For Tank3
  note: Inputs For Tank1
  CT1 : Inport
  F1 : Inport  Port=2
  E1 : Inport  Port=3
  MR1 : Inport  Port=4
  T1 : Inport  Port=5
  EB1 : Inport  Port=6
  CT2 : Inport  Port=7
  F2 : Inport  Port=8
  E2 : Inport  Port=9
  MR2 : Inport  Port=10
  T2 : Inport  Port=11
  EB2 : Inport  Port=12
  Tank1 : Subsystem
  Tank2 : Subsystem
  LL1 : Outport
  LL2 : Outport  Port=2
  wires:
  EB1/1 -> Tank1/6(EB1)
  Tank2/1(LL2) -> LL2/1, Tank1/7(LL2)
  EB2/1 -> Tank2/6(EB2)
  CT2/1 -> Tank2/1(CT2)
  MR1/1 -> Tank1/4(MR1)
  T1/1 -> Tank1/5(T1)
  Tank1/1(LL1) -> LL1/1, Tank2/7(LL1)
  F2/1 -> Tank2/2(F2)
  E2/1 -> Tank2/3(E2)
  F1/1 -> Tank1/2(F1)
  E1/1 -> Tank1/3(E1)
  T2/1 -> Tank2/5(T2)
  CT1/1 -> Tank1/1(CT1)
  MR2/1 -> Tank2/4(MR2)

== system c00003M_harness/M129 ==
  note: VALUES
      | ---------------------------------
      | ControlType = 1 | 2 | 3
      | FillTank = 0 | 1
      | EmptyTank = 0 | 1
      | ManualReference between 0 and 1
      | Tempreature between 0 and 100
      | EmergencyButton = 0 | 1
      | LiquidLevel between 0 and 1 (hmax)
  note: Inputs For Tank2
  note: NAMES
      | --------------------------------------------
      | CT1 = ControlType Tank 1
      | F1 = Fill Tank 1
      | E1 = Empty Tank 1
      | MR1 = Manual Reference Tank1
      | T1 = Temperature Tank 1
      | EB1 = Emergency Button Tank 1
      | LL1 = Liquid Level 1
  note: Inputs For Tank3
  note: Inputs For Tank1
  CT1 : Inport
  F1 : Inport  Port=2
  E1 : Inport  Port=3
  MR1 : Inport  Port=4
  T1 : Inport  Port=5
  EB1 : Inport  Port=6
  CT2 : Inport  Port=7
  F2 : Inport  Port=8
  E2 : Inport  Port=9
  MR2 : Inport  Port=10
  T2 : Inport  Port=11
  EB2 : Inport  Port=12
  Tank1 : Subsystem
  Tank2 : Subsystem
  LL1 : Outport
  LL2 : Outport  Port=2
  wires:
  EB1/1 -> Tank1/6(EB1)
  Tank2/1(LL2) -> LL2/1, Tank1/7(LL2)
  EB2/1 -> Tank2/6(EB2)
  CT2/1 -> Tank2/1(CT2)
  MR1/1 -> Tank1/4(MR1)
  T1/1 -> Tank1/5(T1)
  Tank1/1(LL1) -> LL1/1, Tank2/7(LL1)
  F2/1 -> Tank2/2(F2)
  E2/1 -> Tank2/3(E2)
  F1/1 -> Tank1/2(F1)
  E1/1 -> Tank1/3(E1)
  T2/1 -> Tank2/5(T2)
  CT1/1 -> Tank1/1(CT1)
  MR2/1 -> Tank2/4(MR2)

== system c00003M_harness/M130 ==
  note: VALUES
      | ---------------------------------
      | ControlType = 1 | 2 | 3
      | FillTank = 0 | 1
      | EmptyTank = 0 | 1
      | ManualReference between 0 and 1
      | Tempreature between 0 and 100
      | EmergencyButton = 0 | 1
      | LiquidLevel between 0 and 1 (hmax)
  note: Inputs For Tank2
  note: NAMES
      | --------------------------------------------
      | CT1 = ControlType Tank 1
      | F1 = Fill Tank 1
      | E1 = Empty Tank 1
      | MR1 = Manual Reference Tank1
      | T1 = Temperature Tank 1
      | EB1 = Emergency Button Tank 1
      | LL1 = Liquid Level 1
  note: Inputs For Tank3
  note: Inputs For Tank1
  CT1 : Inport
  F1 : Inport  Port=2
  E1 : Inport  Port=3
  MR1 : Inport  Port=4
  T1 : Inport  Port=5
  EB1 : Inport  Port=6
  CT2 : Inport  Port=7
  F2 : Inport  Port=8
  E2 : Inport  Port=9
  MR2 : Inport  Port=10
  T2 : Inport  Port=11
  EB2 : Inport  Port=12
  Tank1 : Subsystem
  Tank2 : Subsystem
  LL1 : Outport
  LL2 : Outport  Port=2
  wires:
  EB1/1 -> Tank1/6(EB1)
  Tank2/1(LL2) -> LL2/1, Tank1/7(LL2)
  EB2/1 -> Tank2/6(EB2)
  CT2/1 -> Tank2/1(CT2)
  MR1/1 -> Tank1/4(MR1)
  T1/1 -> Tank1/5(T1)
  Tank1/1(LL1) -> LL1/1, Tank2/7(LL1)
  F2/1 -> Tank2/2(F2)
  E2/1 -> Tank2/3(E2)
  F1/1 -> Tank1/2(F1)
  E1/1 -> Tank1/3(E1)
  T2/1 -> Tank2/5(T2)
  CT1/1 -> Tank1/1(CT1)
  MR2/1 -> Tank2/4(MR2)

== system c00003M_harness/M131 ==
  note: VALUES
      | ---------------------------------
      | ControlType = 1 | 2 | 3
      | FillTank = 0 | 1
      | EmptyTank = 0 | 1
      | ManualReference between 0 and 1
      | Tempreature between 0 and 100
      | EmergencyButton = 0 | 1
      | LiquidLevel between 0 and 1 (hmax)
  note: Inputs For Tank2
  note: NAMES
      | --------------------------------------------
      | CT1 = ControlType Tank 1
      | F1 = Fill Tank 1
      | E1 = Empty Tank 1
      | MR1 = Manual Reference Tank1
      | T1 = Temperature Tank 1
      | EB1 = Emergency Button Tank 1
      | LL1 = Liquid Level 1
  note: Inputs For Tank3
  note: Inputs For Tank1
  CT1 : Inport
  F1 : Inport  Port=2
  E1 : Inport  Port=3
  MR1 : Inport  Port=4
  T1 : Inport  Port=5
  EB1 : Inport  Port=6
  CT2 : Inport  Port=7
  F2 : Inport  Port=8
  E2 : Inport  Port=9
  MR2 : Inport  Port=10
  T2 : Inport  Port=11
  EB2 : Inport  Port=12
  Tank1 : Subsystem
  Tank2 : Subsystem
  LL1 : Outport
  LL2 : Outport  Port=2
  wires:
  EB1/1 -> Tank1/6(EB1)
  Tank2/1(LL2) -> LL2/1, Tank1/7(LL2)
  EB2/1 -> Tank2/6(EB2)
  CT2/1 -> Tank2/1(CT2)
  MR1/1 -> Tank1/4(MR1)
  T1/1 -> Tank1/5(T1)
  Tank1/1(LL1) -> LL1/1, Tank2/7(LL1)
  F2/1 -> Tank2/2(F2)
  E2/1 -> Tank2/3(E2)
  F1/1 -> Tank1/2(F1)
  E1/1 -> Tank1/3(E1)
  T2/1 -> Tank2/5(T2)
  CT1/1 -> Tank1/1(CT1)
  MR2/1 -> Tank2/4(MR2)

== system c00003M_harness/M132 ==
  note: VALUES
      | ---------------------------------
      | ControlType = 1 | 2 | 3
      | FillTank = 0 | 1
      | EmptyTank = 0 | 1
      | ManualReference between 0 and 1
      | Tempreature between 0 and 100
      | EmergencyButton = 0 | 1
      | LiquidLevel between 0 and 1 (hmax)
  note: Inputs For Tank2
  note: NAMES
      | --------------------------------------------
      | CT1 = ControlType Tank 1
      | F1 = Fill Tank 1
      | E1 = Empty Tank 1
      | MR1 = Manual Reference Tank1
      | T1 = Temperature Tank 1
      | EB1 = Emergency Button Tank 1
      | LL1 = Liquid Level 1
  note: Inputs For Tank3
  note: Inputs For Tank1
  CT1 : Inport
  F1 : Inport  Port=2
  E1 : Inport  Port=3
  MR1 : Inport  Port=4
  T1 : Inport  Port=5
  EB1 : Inport  Port=6
  CT2 : Inport  Port=7
  F2 : Inport  Port=8
  E2 : Inport  Port=9
  MR2 : Inport  Port=10
  T2 : Inport  Port=11
  EB2 : Inport  Port=12
  Tank1 : Subsystem
  Tank2 : Subsystem
  LL1 : Outport
  LL2 : Outport  Port=2
  wires:
  EB1/1 -> Tank1/6(EB1)
  Tank2/1(LL2) -> LL2/1, Tank1/7(LL2)
  EB2/1 -> Tank2/6(EB2)
  CT2/1 -> Tank2/1(CT2)
  MR1/1 -> Tank1/4(MR1)
  T1/1 -> Tank1/5(T1)
  Tank1/1(LL1) -> LL1/1, Tank2/7(LL1)
  F2/1 -> Tank2/2(F2)
  E2/1 -> Tank2/3(E2)
  F1/1 -> Tank1/2(F1)
  E1/1 -> Tank1/3(E1)
  T2/1 -> Tank2/5(T2)
  CT1/1 -> Tank1/1(CT1)
  MR2/1 -> Tank2/4(MR2)

== system c00003M_harness/M133 ==
  note: VALUES
      | ---------------------------------
      | ControlType = 1 | 2 | 3
      | FillTank = 0 | 1
      | EmptyTank = 0 | 1
      | ManualReference between 0 and 1
      | Tempreature between 0 and 100
      | EmergencyButton = 0 | 1
      | LiquidLevel between 0 and 1 (hmax)
  note: Inputs For Tank2
  note: NAMES
      | --------------------------------------------
      | CT1 = ControlType Tank 1
      | F1 = Fill Tank 1
      | E1 = Empty Tank 1
      | MR1 = Manual Reference Tank1
      | T1 = Temperature Tank 1
      | EB1 = Emergency Button Tank 1
      | LL1 = Liquid Level 1
  note: Inputs For Tank3
  note: Inputs For Tank1
  CT1 : Inport
  F1 : Inport  Port=2
  E1 : Inport  Port=3
  MR1 : Inport  Port=4
  T1 : Inport  Port=5
  EB1 : Inport  Port=6
  CT2 : Inport  Port=7
  F2 : Inport  Port=8
  E2 : Inport  Port=9
  MR2 : Inport  Port=10
  T2 : Inport  Port=11
  EB2 : Inport  Port=12
  Tank1 : Subsystem
  Tank2 : Subsystem
  LL1 : Outport
  LL2 : Outport  Port=2
  wires:
  EB1/1 -> Tank1/6(EB1)
  Tank2/1(LL2) -> LL2/1, Tank1/7(LL2)
  EB2/1 -> Tank2/6(EB2)
  CT2/1 -> Tank2/1(CT2)
  MR1/1 -> Tank1/4(MR1)
  T1/1 -> Tank1/5(T1)
  Tank1/1(LL1) -> LL1/1, Tank2/7(LL1)
  F2/1 -> Tank2/2(F2)
  E2/1 -> Tank2/3(E2)
  F1/1 -> Tank1/2(F1)
  E1/1 -> Tank1/3(E1)
  T2/1 -> Tank2/5(T2)
  CT1/1 -> Tank1/1(CT1)
  MR2/1 -> Tank2/4(MR2)

== system c00003M_harness/M134 ==
  note: VALUES
      | ---------------------------------
      | ControlType = 1 | 2 | 3
      | FillTank = 0 | 1
      | EmptyTank = 0 | 1
      | ManualReference between 0 and 1
      | Tempreature between 0 and 100
      | EmergencyButton = 0 | 1
      | LiquidLevel between 0 and 1 (hmax)
  note: Inputs For Tank2
  note: NAMES
      | --------------------------------------------
      | CT1 = ControlType Tank 1
      | F1 = Fill Tank 1
      | E1 = Empty Tank 1
      | MR1 = Manual Reference Tank1
      | T1 = Temperature Tank 1
      | EB1 = Emergency Button Tank 1
      | LL1 = Liquid Level 1
  note: Inputs For Tank3
  note: Inputs For Tank1
  CT1 : Inport
  F1 : Inport  Port=2
  E1 : Inport  Port=3
  MR1 : Inport  Port=4
  T1 : Inport  Port=5
  EB1 : Inport  Port=6
  CT2 : Inport  Port=7
  F2 : Inport  Port=8
  E2 : Inport  Port=9
  MR2 : Inport  Port=10
  T2 : Inport  Port=11
  EB2 : Inport  Port=12
  Tank1 : Subsystem
  Tank2 : Subsystem
  LL1 : Outport
  LL2 : Outport  Port=2
  wires:
  EB1/1 -> Tank1/6(EB1)
  Tank2/1(LL2) -> LL2/1, Tank1/7(LL2)
  EB2/1 -> Tank2/6(EB2)
  CT2/1 -> Tank2/1(CT2)
  MR1/1 -> Tank1/4(MR1)
  T1/1 -> Tank1/5(T1)
  Tank1/1(LL1) -> LL1/1, Tank2/7(LL1)
  F2/1 -> Tank2/2(F2)
  E2/1 -> Tank2/3(E2)
  F1/1 -> Tank1/2(F1)
  E1/1 -> Tank1/3(E1)
  T2/1 -> Tank2/5(T2)
  CT1/1 -> Tank1/1(CT1)
  MR2/1 -> Tank2/4(MR2)
